simulink library "lib_GenHeatX_LumpedMassHeatX"  (R2015a)
settings: Solver=ode45  StartTime=0.0  StopTime=10.0  RelTol=1e-3
settings Model: Creator=jlkratz  LastModifiedBy=jlkratz

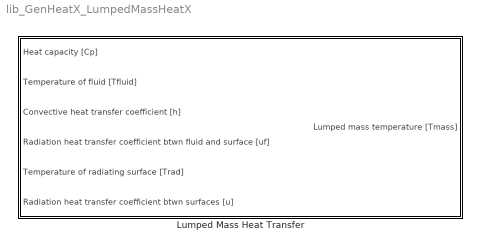
== system lib_GenHeatX_LumpedMassHeatX ==
  Lumped Mass Heat Transfer : Subsystem  mask(TSAT: Lumped Mass Heat Transfer Block){Tmass0_M=500, m_M=1, conv_M=on, radf_M=on, Aconv_M=0.5, rads_M=on, Arad_M=0.5}
      mask prompts: Tmass0_M "Tmass0_M - Initial temperature"; m_M "m_M - Mass"; conv_M "conv_M - Consider convection?"; radf_M "radf_M - Consider radiation with the fluid?"; Aconv_M "Aconv_M - Effective area for convective heat transfer"; rads_M "rads_M - Consider radiation with external surfaces?"; Arad_M "Arad_M - Effective area for radiation heat transfer"
      mask help: This function simulates heat transfer of a structural component which can be appropriately modeled as a lumped mass. See the block help menu for guidelines. The block attempts to address heat transfer due to convection with a fluid but also has options that attempt to consider radiation to the fluid as well as external surfaces. Definitions for the heat transfer coefficients are provided in the help menu.
      mask init:
      | % inport and constant block swapping -------------------------------------%
      | 
      | % Inport Numbers
      | n = 2; %first inport number
      | 
      | % Fluid Temperature Inport
      | if conv_M == 1 || radf_M == 1
      |     if strcmp(get_param([gcb '/Temperature of fluid [Tfluid]'],'BlockType'),'Constant')
      |         MSK_ReplaceBlock_TMATS([gcb '/Temperature of fluid [Tfluid]'],'built-in/Inport');
      |     end
      |     set_param([gcb '/Temperature of fluid [Tfluid]'],'Port',num2str(n));
      |     n = n + 1;
      | else
      |     if strcmp(get_param([gcb '/Temperature of fluid [Tfluid]'],'BlockType'),'Inport')
      |         MSK_ReplaceBlock_TMATS([gcb '/Temperature of fluid [Tfluid]'],'built-in/Constant');
      |         set_param([gcb '/Temperature of fluid [Tfluid]'],'Value','0');
      |     end
      | end
      | 
      | % Fluid Convection Inport
      | if conv_M == 1
      |     if strcmp(get_param([gcb '/Convective heat transfer coefficient [h]'],'BlockType'),'Constant')
      |         MSK_ReplaceBlock_TMATS([gcb '/Convective heat transfer coefficient [h]'],'built-in/Inport');
      |     end
      |     set_param([gcb '/Convective heat transfer coefficient [h]'],'Port',num2str(n));
      |     n = n + 1;
      | else
      |     if strcmp(get_param([gcb '/Convective heat transfer coefficient [h]'],'BlockType'),'Inport')
      |         MSK_ReplaceBlock_TMATS([gcb '/Convective heat transfer coefficient [h]'],'built-in/Constant');
      |         set_param([gcb '/Convective heat transfer coefficient [h]'],'Value','0');
      |     end
      | end
      | 
      | % Radiation with Fluid
      | if radf_M == 1
      |     if strcmp(get_param([gcb '/Radiation heat transfer coefficient btwn fluid and surface [uf]'],'BlockType'),'Constant')
      |         MSK_ReplaceBlock_TMATS([gcb '/Radiation heat transfer coefficient btwn fluid and surface [uf]'],'built-in/Inport');
      |     end
      |     set_param([gcb '/Radiation heat transfer coefficient btwn fluid and surface [uf]'],'Port',num2str(n));
      |     n = n + 1;
      | else
      |     if strcmp(get_param([gcb '/Radiation heat transfer coefficient btwn fluid and surface [uf]'],'BlockType'),'Inport')
      |         MSK_ReplaceBlock_TMATS([gcb '/Radiation heat transfer coefficient btwn fluid and surface [uf]'],'built-in/Constant');
      |         set_param([gcb '/Radiation heat transfer coefficient btwn fluid and surface [uf]'],'Value','0');
      |     end
      | end
      | 
      | % Radiation with Surfaces
      | if rads_M == 1
      |     if strcmp(get_param([gcb '/Temperature of radiating surface [Trad]'],'BlockType'),'Constant')
      |         MSK_ReplaceBlock_TMATS([gcb '/Temperature of radiating surface [Trad]'],'built-in/Inport');
      |         MSK_ReplaceBlock_TMATS([gcb '/Radiation heat transfer coefficient btwn surfaces [u]'],'built-in/Inport');
      |     end
      |     set_param([gcb '/Temperature of radiating surface [Trad]'],'Port',num2str(n));
      |     set_param([gcb '/Radiation heat transfer coefficient btwn surfaces [u]'],'Port',num2str(n+1));
      |     n = n + 2;
      | else
      |     if strcmp(get_param([gcb '/Temperature of radiating surface [Trad]'],'BlockType'),'Inport')
      |         MSK_ReplaceBlock_TMATS([gcb '/Temperature of radiating surface [Trad]'],'built-in/Constant');
      |         MSK_ReplaceBlock_TMATS([gcb '/Radiation heat transfer coefficient btwn surfaces [u]'],'built-in/Constant');
      |         set_param([gcb '/Temperature of radiating surface [Trad]'],'Value','0');
      |         set_param([gcb '/Radiation heat transfer coefficient btwn surfaces [u]'],'Value','0');
      |     end
      | end
      mask Help: web(which('GenHeatX_TSAT_LumpedMassHeatX.html'),'-helpbrowser')
      mask Callback conv_M:
      | if length(get_param(gcb,'conv_M')) == 2 %on
      |     if length(get_param(gcb,'radf_M')) ~= 2
      |         MSK_SEC_Enables_TMATS('conv_M',5,'en')
      |     end
      | else
      |     if length(get_param(gcb,'radf_M')) ~= 2
      |         MSK_SEC_Enables_TMATS('conv_M',5,'en')
      |     end
      | end
      mask Callback radf_M:
      | if length(get_param(gcb,'radf_M')) == 2 %on
      |     if length(get_param(gcb,'conv_M')) ~= 2
      |         MSK_SEC_Enables_TMATS('radf_M',5,'en')
      |     end
      | else
      |     if length(get_param(gcb,'conv_M')) ~= 2
      |         MSK_SEC_Enables_TMATS('radf_M',5,'en')
      |     end
      | end
      mask Callback rads_M:
      | MSK_SEC_Enables_TMATS('rads_M',7,'en')
      | % if length(get_param(gcb,'radf_M'))%on
      | %     if length(get_param(gcb,'rads_M')) ~= 2
      | %         MSK_SEC_Enables_TMATS('radf_M',7,'en')
      | %     end
      | % else
      | %     if length(get_param(gcb,'rads_M')) ~= 2
      | %         MSK_SEC_Enables_TMATS('radf_M',7,'en')
      | %     end
      | % end
      mask DialogControl Container3 Prompt: Heat transfer from a fluid
      mask DialogControl Container5 Prompt: Heat transfer from external surfaces

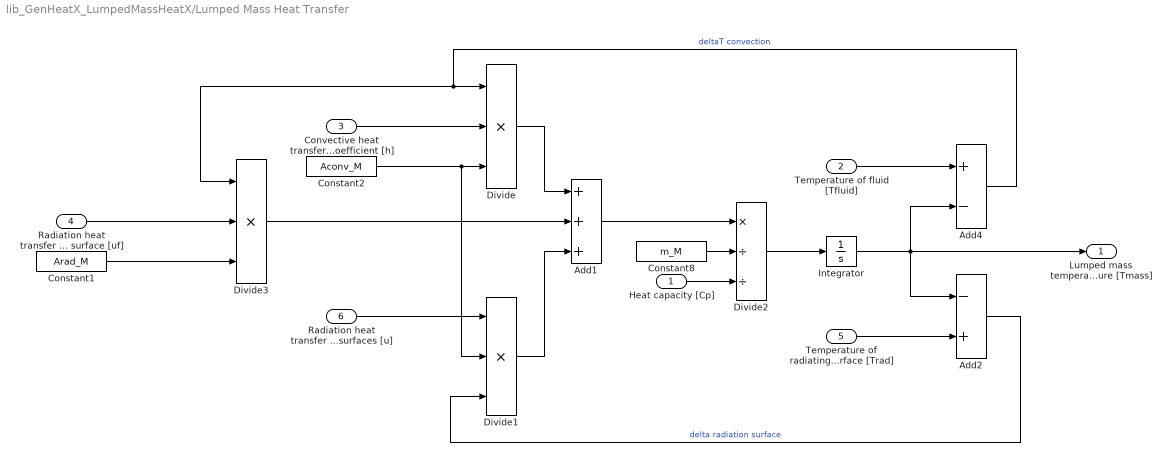
== system lib_GenHeatX_LumpedMassHeatX/Lumped Mass Heat Transfer ==
  Heat capacity [Cp] : Inport
  Temperature of fluid [Tfluid] : Inport  Port=2
  Convective heat transfer coefficient [h] : Inport  Port=3
  Radiation heat transfer coefficient btwn fluid and surface [uf] : Inport  Port=4
  Temperature of radiating surface [Trad] : Inport  Port=5
  Radiation heat transfer coefficient btwn surfaces [u] : Inport  Port=6
  Add1 : Sum  Inputs=+++
  Add2 : Sum  Inputs=-+
  Add4 : Sum  Inputs=+-
  Constant1 : Constant  Value=Arad_M
  Constant2 : Constant  Value=Aconv_M
  Constant8 : Constant  Value=m_M
  Divide : Product  Inputs=***
  Divide1 : Product  Inputs=***
  Divide2 : Product  Inputs=*//
  Divide3 : Product  Inputs=***
  Integrator : Integrator  InitialCondition=Tmass0_M
  Lumped mass temperature [Tmass] : Outport
  wires:
  Divide3/1 -> Add1/2
  Radiation heat transfer coefficient btwn fluid and surface [uf]/1 -> Divide3/2
  Constant1/1 -> Divide3/3
  Divide1/1 -> Add1/3
  Convective heat transfer coefficient [h]/1 -> Divide/2
  Divide/1 -> Add1/1
  Radiation heat transfer coefficient btwn surfaces [u]/1 -> Divide1/1
  Divide2/1 -> Integrator/1
  Heat capacity [Cp]/1 -> Divide2/3
  Integrator/1 -> Add4/2, Add2/1, Lumped mass temperature [Tmass]/1
  Add1/1 -> Divide2/1
  Constant8/1 -> Divide2/2
  Add2/1 -> Divide1/3  "delta radiation surface"
  Constant2/1 -> Divide/3, Divide1/2
  Temperature of radiating surface [Trad]/1 -> Add2/2
  Temperature of fluid [Tfluid]/1 -> Add4/1
  Add4/1 -> Divide/1, Divide3/1  "deltaT convection"
